simulink model "tests"  (R2024b)
settings: Solver=VariableStepAuto  StartTime=0.0  StopTime=1  RelTol=1e-3  AbsTol=1e-3  EnableMultiTasking=on
values from neighbouring files (symbols this model uses):
  m = obj.Br *obj.volume / obj.mu    [External_Magnet2.m]
  N = gridSizes(k)    [Test.m]
  Params = Sim_Param_Setup    [Sim_Open.m]
undefined symbols (not defined in the file or in its folder): X, Y, Z
libraries: sm_lib x88, vrlib x72, nesl_utility x52, matrix_library x46, sharedtransform x6
(part 5 of 5)

== matlab function tests/Subsystem/Single_Arm/Plate_1/Torques and Forces/Magnetic Torques/MATLAB Function ==
  data: r2 input; M2 input; u input; y output; Params input
function y = fcn(r2, M2, u, Params)

coords_w = linspace(-Params.LinkWidth/2 + Params.LinkWidth/(2*Params.N), Params.LinkWidth/2 - Params.LinkWidth/(2*Params.N), Params.N);
coords_l = linspace(-Params.LinkLength/2 + Params.LinkLength/(2*Params.N), Params.LinkLength/2 - Params.LinkLength/(2*Params.N), Params.N);
m_vec = M2 / (Params.N^2);

Bn = zeros(3,1);

for i=1:Params.N
    for j=1:Params.N

        offset = [coords_w(j); 0; coords_l(i)];
        r_vec = r2 - u*offset;
        r_hat = r_vec / norm(r_vec);

        B = Params.mu/(4*pi*norm(r_vec)^3) * (3*(r_hat*r_hat') - eye(3)) * m_vec;

        Bn = Bn + B;

    end
end

y = Bn;

== matlab function tests/Subsystem/Single_Arm/Plate_6/Torques and Forces/Magnetic Torques/MATLAB Function ==
  data: r5 input; M5 input; u input; y output; Params input
function y = fcn(r5, M5, u, Params)


w = [-Params.LinkWidth/2+Params.LinkWidth/(2*Params.N); 0; -Params.LinkLength/2+Params.LinkLength/(2*Params.N)];
m_vec = M5 / Params.N^2;

Bn = zeros(3,1);

for i=1:Params.N
    for j=1:Params.N

        offset = [Params.LinkWidth*(i-1)/Params.N; 0; Params.LinkLength*(j-1)/Params.N];
        w_vec = w+offset;
        r_vec = r5 - u*w_vec;
        r_hat = r_vec / norm(r_vec);

        B = Params.mu/(4*pi*norm(r_vec)^3) * (3*(r_hat*r_hat') - eye(3)) * m_vec;

        Bn = Bn + B;

    end
end

y = Bn;

== matlab function tests/Subsystem/Single_Arm/Plate_2/Torques and Forces/Magnetic Torques/MATLAB Function ==
  data: r1 input; M1 input; u input; y output; Params input
function y = fcn(r1, M1, u, Params)

coords_w = linspace(-Params.LinkWidth/2 + Params.LinkWidth/(2*Params.N), Params.LinkWidth/2 - Params.LinkWidth/(2*Params.N), Params.N);
coords_l = linspace(-Params.LinkLength/2 + Params.LinkLength/(2*Params.N), Params.LinkLength/2 - Params.LinkLength/(2*Params.N), Params.N);
m_vec = M1 / (Params.N^2);

Bn = zeros(3,1);

for i=1:Params.N
    for j=1:Params.N

        offset = [coords_w(j); 0; coords_l(i)];
        r_vec = r1 - u*offset;
        r_hat = r_vec / norm(r_vec);

        B = Params.mu/(4*pi*norm(r_vec)^3) * (3*(r_hat*r_hat') - eye(3)) * m_vec;

        Bn = Bn + B;

    end
end

y = Bn;

== matlab function tests/Subsystem/Single_Arm/Plate_2/Torques and Forces/Magnetic Torques/MATLAB Function1 ==
  data: r3 input; M3 input; u input; y output; Params input
function y = fcn(r3, M3, u, Params)

coords_w = linspace(-Params.LinkWidth/2 + Params.LinkWidth/(2*Params.N), Params.LinkWidth/2 - Params.LinkWidth/(2*Params.N), Params.N);
coords_l = linspace(-Params.LinkLength/2 + Params.LinkLength/(2*Params.N), Params.LinkLength/2 - Params.LinkLength/(2*Params.N), Params.N);
m_vec = M3 / (Params.N^2);

Bn = zeros(3,1);

for i=1:Params.N
    for j=1:Params.N

        offset = [coords_w(j); 0; coords_l(i)];
        r_vec = r3 - u*offset;
        r_hat = r_vec / norm(r_vec);

        B = Params.mu/(4*pi*norm(r_vec)^3) * (3*(r_hat*r_hat') - eye(3)) * m_vec;

        Bn = Bn + B;

    end
end

y = Bn;

== matlab function tests/Subsystem/Single_Arm/Plate_3/Torques and Forces/Magnetic Torques/MATLAB Function ==
  data: M2 input; r2 input; u input; y output; Params input
function y = fcn(M2, r2, u, Params)

coords_w = linspace(-Params.LinkWidth/2 + Params.LinkWidth/(2*Params.N), Params.LinkWidth/2 - Params.LinkWidth/(2*Params.N), Params.N);
coords_l = linspace(-Params.LinkLength/2 + Params.LinkLength/(2*Params.N), Params.LinkLength/2 - Params.LinkLength/(2*Params.N), Params.N);
m_vec = M2 / (Params.N^2);

Bn = zeros(3,1);

for i=1:Params.N
    for j=1:Params.N

        offset = [coords_w(j); 0; coords_l(i)];
        r_vec = r2 - u*offset;
        r_hat = r_vec / norm(r_vec);

        B = Params.mu/(4*pi*norm(r_vec)^3) * (3*(r_hat*r_hat') - eye(3)) * m_vec;

        Bn = Bn + B;

    end
end

y = Bn;

== matlab function tests/Subsystem/Single_Arm/Plate_3/Torques and Forces/Magnetic Torques/MATLAB Function1 ==
  data: M4 input; r4 input; u input; y output; Params input
function y = fcn(M4, r4, u, Params)

coords_w = linspace(-Params.LinkWidth/2 + Params.LinkWidth/(2*Params.N), Params.LinkWidth/2 - Params.LinkWidth/(2*Params.N), Params.N);
coords_l = linspace(-Params.LinkLength/2 + Params.LinkLength/(2*Params.N), Params.LinkLength/2 - Params.LinkLength/(2*Params.N), Params.N);
m_vec = M4 / (Params.N^2);

Bn = zeros(3,1);

for i=1:Params.N
    for j=1:Params.N

        offset = [coords_w(j); 0; coords_l(i)];
        r_vec = r4 - u*offset;
        r_hat = r_vec / norm(r_vec);

        B = Params.mu/(4*pi*norm(r_vec)^3) * (3*(r_hat*r_hat') - eye(3)) * m_vec;

        Bn = Bn + B;

    end
end

y = Bn;

== matlab function tests/Subsystem/Single_Arm/Plate_4/Torques and Forces/Magnetic Torques/MATLAB Function1 ==
  data: M3 input; r3 input; u input; y output; Params input
function y = fcn(M3, r3, u, Params)

coords_w = linspace(-Params.LinkWidth/2 + Params.LinkWidth/(2*Params.N), Params.LinkWidth/2 - Params.LinkWidth/(2*Params.N), Params.N);
coords_l = linspace(-Params.LinkLength/2 + Params.LinkLength/(2*Params.N), Params.LinkLength/2 - Params.LinkLength/(2*Params.N), Params.N);
m_vec = M3 / (Params.N^2);

Bn = zeros(3,1);

for i=1:Params.N
    for j=1:Params.N

        offset = [coords_w(j); 0; coords_l(i)];
        r_vec = r3 - u*offset;
        r_hat = r_vec / norm(r_vec);

        B = Params.mu/(4*pi*norm(r_vec)^3) * (3*(r_hat*r_hat') - eye(3)) * m_vec;

        Bn = Bn + B;

    end
end

y = Bn;

== matlab function tests/Subsystem/Single_Arm/Plate_4/Torques and Forces/Magnetic Torques/MATLAB Function2 ==
  data: M5 input; r5 input; u input; y output; Params input
function y = fcn(M5, r5, u, Params)

coords_w = linspace(-Params.LinkWidth/2 + Params.LinkWidth/(2*Params.N), Params.LinkWidth/2 - Params.LinkWidth/(2*Params.N), Params.N);
coords_l = linspace(-Params.LinkLength/2 + Params.LinkLength/(2*Params.N), Params.LinkLength/2 - Params.LinkLength/(2*Params.N), Params.N);
m_vec = M5 / (Params.N^2);

Bn = zeros(3,1);

for i=1:Params.N
    for j=1:Params.N

        offset = [coords_w(j); 0; coords_l(i)];
        r_vec = r5 - u*offset;
        r_hat = r_vec / norm(r_vec);

        B = Params.mu/(4*pi*norm(r_vec)^3) * (3*(r_hat*r_hat') - eye(3)) * m_vec;

        Bn = Bn + B;

    end
end

y = Bn;

== matlab function tests/Subsystem/Single_Arm/Plate_5/Torques and Forces/Magnetic Torques/MATLAB Function2 ==
  data: M4 input; r4 input; u input; y output; Params input
function y = fcn(M4, r4, u, Params)

coords_w = linspace(-Params.LinkWidth/2 + Params.LinkWidth/(2*Params.N), Params.LinkWidth/2 - Params.LinkWidth/(2*Params.N), Params.N);
coords_l = linspace(-Params.LinkLength/2 + Params.LinkLength/(2*Params.N), Params.LinkLength/2 - Params.LinkLength/(2*Params.N), Params.N);
m_vec = M4 / (Params.N^2);

Bn = zeros(3,1);

for i=1:Params.N
    for j=1:Params.N

        offset = [coords_w(j); 0; coords_l(i)];
        r_vec = r4 - u*offset;
        r_hat = r_vec / norm(r_vec);

        B = Params.mu/(4*pi*norm(r_vec)^3) * (3*(r_hat*r_hat') - eye(3)) * m_vec;

        Bn = Bn + B;

    end
end

y = Bn;
